simulink model "DAB_OpenLoop"  (R2024a)
settings: Solver=ode23t  StartTime=0.0  StopTime=10.0  RelTol=1e-3
libraries: spsMosfetLib x8, spsSeriesRLCBranchLib x3, spsVoltageMeasurementLib x3, spsCurrentMeasurementLib x1, spsDCVoltageSourceLib x1, spsLinearTransformerLib x1, sps_lib x1
settings Model: Creator=User  LastModifiedBy=User

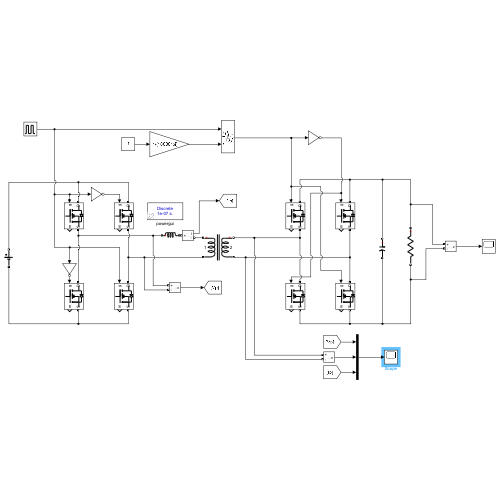
[thumbnail: Simulink's stored preview of the top-level diagram]
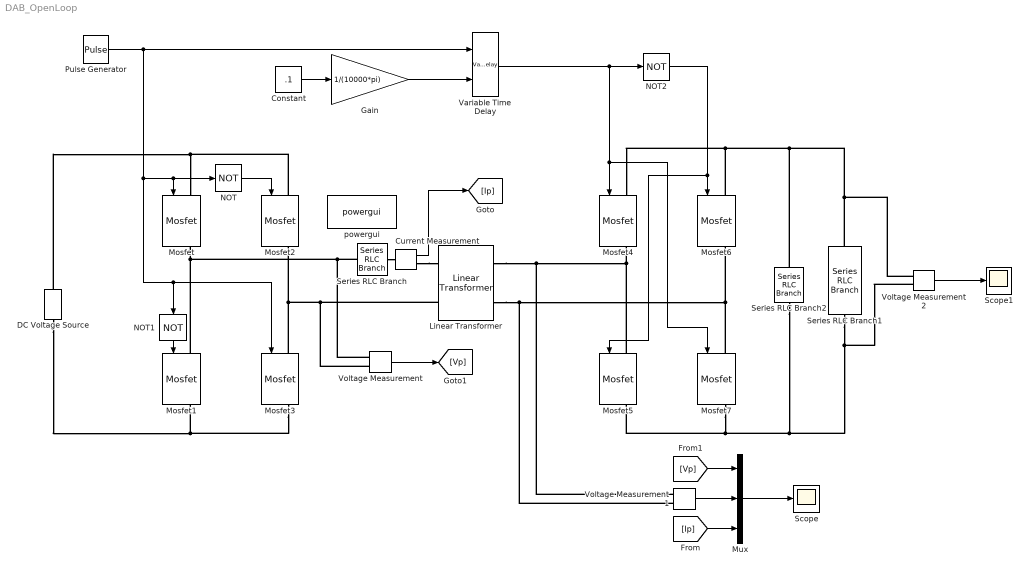
== system DAB_OpenLoop ==
  Constant : Constant  Value=.1
  Current Measurement : spsCurrentMeasurementLib/Current Measurement  PhasorSimulation=off  OutputType=Complex  PSBequivalent=0
  DC Voltage Source : spsDCVoltageSourceLib/DC Voltage Source  Amplitude=1000  Measurements=None
  Gain : Gain  Gain=1/(10000*pi)
  Linear Transformer : spsLinearTransformerLib/Linear Transformer  UNITS=SI  NominalPower=[ 250e6 10000*pi ]  winding1=[500 0 0]  winding2=[250 0 0]  ThreeWindings=off  winding3=[3.15e+05 0.7938 0.084225]  RmLm=[1.0804e+06 2866]  Measurements=None  DataType=on
  Mosfet{,1..7} (8 alike) : spsMosfetLib/Mosfet  Ron=0.1  Lon=0  Rd=0.01  Vfd=0  IC=0  Rs=1e5  Cs=inf  Measurements=on
  Mux : Mux  Inputs=3
  NOT : Logic  Operator=NOT  IconShape=distinctive  AllPortsSameDT=off  OutDataTypeStr=boolean
  NOT1 : Logic  Operator=NOT  IconShape=distinctive  AllPortsSameDT=off  OutDataTypeStr=boolean
  NOT2 : Logic  Operator=NOT  IconShape=distinctive  AllPortsSameDT=off  OutDataTypeStr=boolean
  Pulse Generator : DiscretePulseGenerator  PulseType=Time based  Period=1/(10000*pi)  PulseWidth=50
  Scope : Scope
  Scope1 : Scope
  Series RLC Branch : spsSeriesRLCBranchLib/Series RLC Branch  LConnTagsString=__new0  RConnTagsString=__new0  BranchType=L  Resistance=1  Inductance=.0102e-3  SetiL0=off  InitialCurrent=0  Capacitance=1e-6  Setx0=off  InitialVoltage=0  Measurements=None
  Series RLC Branch1 : spsSeriesRLCBranchLib/Series RLC Branch  LConnTagsString=__new0  RConnTagsString=__new0  BranchType=R  Resistance=1  Inductance=1e-3  SetiL0=off  InitialCurrent=0  Capacitance=1e-6  Setx0=off  InitialVoltage=0  Measurements=None
  Series RLC Branch2 : spsSeriesRLCBranchLib/Series RLC Branch  LConnTagsString=__new0  RConnTagsString=__new0  BranchType=C  Resistance=1  Inductance=1e-3  SetiL0=off  InitialCurrent=0  Capacitance=660e-6  Setx0=off  InitialVoltage=0  Measurements=None
  Variable Time Delay : VariableTransportDelay  MaximumDelay=10
  Voltage Measurement : spsVoltageMeasurementLib/Voltage Measurement  PhasorSimulation=off  OutputType=Complex  PSBequivalent=0
  Voltage Measurement1 : spsVoltageMeasurementLib/Voltage Measurement  PhasorSimulation=off  OutputType=Complex  PSBequivalent=0
  Voltage Measurement2 : spsVoltageMeasurementLib/Voltage Measurement  PhasorSimulation=off  OutputType=Complex  PSBequivalent=0
  powergui : sps_lib/powergui  Priority=1  SimulationMode=Discrete  SampleTime=1e-7  frequency=60  Iterations=50  frequencyindice=0  Pbase=100e6  ErrMax=1e-4  UnitsV=kV  UnitsW=MW  buscounter=0  FunctionMessages=off  echomessages=off  EnableUseOfTLC=off  CurrentSourceSwitches=off  DisableSnubberDevices=off  DisableRonSwitches=off  DisableVfSwitches=off  DisplayEquations=off  AutomaticDiscreteSolvers=off  SolverType=Tustin/Backward Euler (TBE)  Interpol=off  ExternalGateDelay=off  methode=off  Ts=100  x0status=blocks  SPID=on  SwTol=0  HookPort=off  NonlinearTolerance=1e-4  nMaxIteration=100  ContinueOnMaxIteration=off  RestoreLinks=warning  ResistiveCurrentMeasurement=off  Frange=[0:2:500]  Ylog=off  Xlog=on  ShowGrid=off  save=off  variable=ZData  structure=0  ZoomFFT=off  StartTime=0.0  cycles=1  DisplayStyle=1  fundamental=60  FreqAxis=off  MaxFrequency=1000  frequencyindicesteady=1  RmsSteady=1  display=off
  wires:
  Current Measurement/1 -> [Ip]
  Voltage Measurement/1 -> [Vp]
  [Vp] -> Mux/1
  Voltage Measurement1/1 -> Mux/2
  [Ip] -> Mux/3
  Mux/1 -> Scope/1
  Voltage Measurement2/1 -> Scope1/1
  NOT/1 -> Mosfet2/1
  NOT1/1 -> Mosfet1/1
  Pulse Generator/1 -> NOT1/1, Mosfet3/1, NOT/1, Mosfet/1, Variable Time Delay/1
  Constant/1 -> Gain/1
  Gain/1 -> Variable Time Delay/2
  Variable Time Delay/1 -> NOT2/1, Mosfet7/1, Mosfet4/1
  NOT2/1 -> Mosfet5/1, Mosfet6/1
  connections:
  Mosfet1/LConn1 -- Voltage Measurement/LConn1 -- Series RLC Branch/LConn1 -- Mosfet/RConn1
  Mosfet3/LConn1 -- Voltage Measurement/LConn2 -- Linear Transformer/LConn2 -- Mosfet2/RConn1
  Mosfet2/LConn1 -- DC Voltage Source/RConn1 -- Mosfet/LConn1
  Mosfet3/RConn1 -- DC Voltage Source/LConn1 -- Mosfet1/RConn1
  Mosfet7/RConn1 -- Voltage Measurement2/LConn2 -- Series RLC Branch1/RConn1 -- Series RLC Branch2/RConn1 -- Mosfet5/RConn1
  Mosfet6/LConn1 -- Voltage Measurement2/LConn1 -- Series RLC Branch1/LConn1 -- Series RLC Branch2/LConn1 -- Mosfet4/LConn1
  Mosfet7/LConn1 -- Voltage Measurement1/LConn2 -- Linear Transformer/RConn2 -- Mosfet6/RConn1
  Mosfet5/LConn1 -- Voltage Measurement1/LConn1 -- Linear Transformer/RConn1 -- Mosfet4/RConn1
  Current Measurement/RConn1 -- Linear Transformer/LConn1
  Series RLC Branch/RConn1 -- Current Measurement/LConn1
